simulink model "LeTronJames_Assignment2"  (R2022a)
settings: Solver=FixedStepAuto  StartTime=0.0  StopTime=60.0  FixedStep=1e-3  RelTol=1e-3  EnableMultiTasking=on
undefined symbols (not defined in the file): A0, A1, D0, D1, D10, D11, D12, D13, D2, D3, D4, D5, D6, D7, D8, D9, magnitude, PTA0, PTA1, PTA2, PTB2, PTB23, PTB3, PTB9, PTC16, PTC17, PTC2, PTC3, PTC4, PTD0, PTD1, PTD2, PTD3
libraries: frdmk64flib x19, etargetslib x2
settings Model: ExtModeTrigDuration=5  Creator=vinee  LastModifiedBy=yajatsharma
settings SolverCC: AlgebraicLoopSolver=TrustRegion
settings OptimizationCC: EnhancedBackFolding=on  PassReuseOutputArgsAs=Individual arguments  ZeroExternalMemoryAtStartup=off  ZeroInternalMemoryAtStartup=off  MaxStackSize=64  OptimizeBlockOrder=speed  DifferentSizesBufferReuse=on  OptimizationCustomize=off  EfficientTunableParamExpr=on
settings DebuggingCC: ParameterTunabilityLossMsg=error  UnconnectedInputMsg=warning  UnconnectedOutputMsg=warning  UnconnectedLineMsg=warning  SFMachineParentedDataDiag=warning
settings HardwareCC: ProdBitPerPointer=32  ProdBitPerSizeT=32  ProdBitPerPtrDiffT=32  ProdLargestAtomicInteger=Long  ProdLargestAtomicFloat=Double  ProdWordSize=32  ProdHWDeviceType=ARM Compatible->ARM Cortex
settings SFSimCC: MATLABDynamicMemAlloc=off
settings RTWCC: SystemTargetFile=ert.tlc  HardwareBoard=NXP FRDM-K64F  TLCOptions="-aInlineSetEventsForThisBaseRateFcn=TLC_FALSE -aSuppressMultiTaskScheduler=TLC_FALSE  -aRateBasedStepFcn=0"  TemplateMakefile=ert_default_tmf  Toolchain=GNU Tools for ARM Embedded Processors
settings CodeAppCC: ForceParamTrailComments=on  IgnoreCustomStorageClasses=off  OperatorAnnotations=on  SimulinkDataObjDesc=on  SFDataObjDesc=on  InsertBlockDesc=on

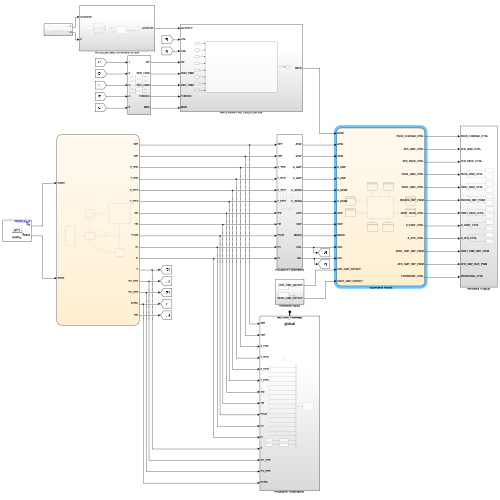
[thumbnail: Simulink's stored preview of the top-level diagram]
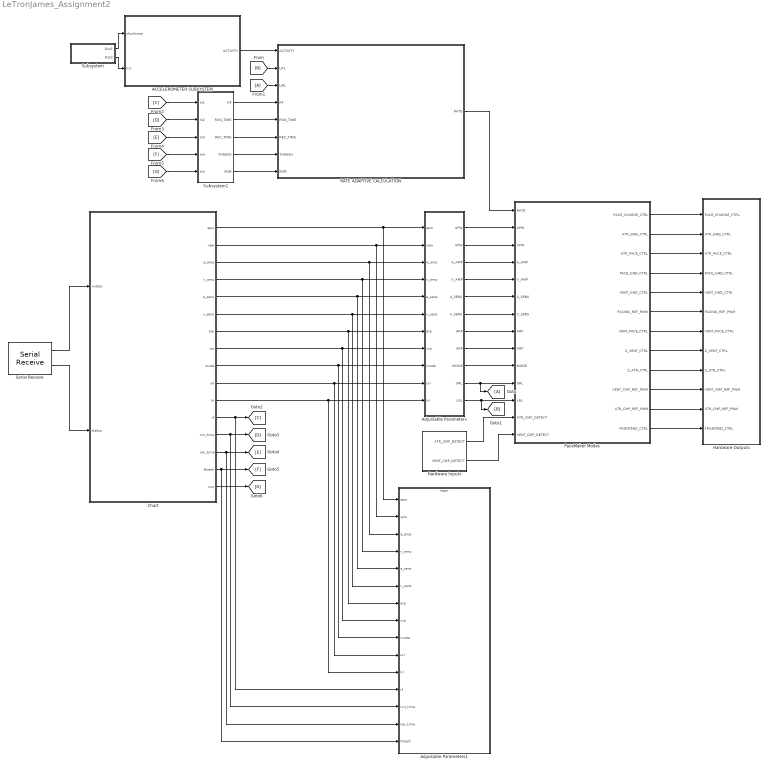
== system LeTronJames_Assignment2 ==
  ACCELEROMETER SUBSYSTEM : Subsystem
  Adjustable Parameters : Subsystem
  Adjustable Parameters1 : Subsystem
  Chart : Stateflow chart  TreatAsAtomicUnit=on
  From1 : From
  Goto : Goto
  Hardware Inputs : Subsystem
  Hardware Outputs : Subsystem
  PaceMaker Modes : Stateflow chart  TreatAsAtomicUnit=on
      settings: PortSchema="{\"entries\":[{\"content\":{\"sides\":[{\"content\":{\"connectorIds\":[\"In14\",\"In1\",\"In4\",\"In2\",\"In3\",\"In5\",\"In6\",\"In7\",\"In8\",\"In9\",\"In13\",\"In11\",\"In12\",\"In10\"]},\"type\":\"ConnectorPlacement.EquallySpacedRectSide\",\"uuid\":\"77d3ccf4-73ab-4fa0-a75b-8c1b7a05e3d5\"},{\"content\":{\"connectorIds\":[\"Out1\",\"Out2\",\"Out3\",\"Out4\",\"Out5\",\"Out6\",\"Out7\",\"Out8\",\"Out9\",\"Out10\",\"Out11\",\"Out12\"],\"side\":\"RIGHT\"},\"type\":\"ConnectorPlacement.EquallySpacedRectSide\",\"uuid\":\"3fd88102-4650-4f47-a7ab-d0892a3e0c85\"},{\"content\":{\"connectorIds\":[],\"side\":\"TOP\"},\"type\":\"ConnectorPlacement.EquallySpacedRectSide\",\"uuid\":\"24053871-acf1-4df3-bb57-3135065b83a4\"}]},\"type\":\"ConnectorPlacement.EquallySpacedConnector\",\"uuid\":\"a590c136-0049-4ce2-946f-1a46cb69b8d2\"}],\"packageUris\":[\"http://schema.mathworks.com/mf0/Connector/R2020b\"],\"version\":\"1.0\"}"
  RATE ADAPTIVE CALCULATION : Subsystem
  Serial Receive : frdmk64flib/Serial Receive  SCIModule=0  Baudrate=uint32(9600)  Parity=None  StopBits=1  HardwareFlowControl=None  ByteOrder=LittleEndian  DataType=uint8  DataLength=17  BlockingMode=off  OutputStatus=on  SampleTime=-1
  Subsystem : Subsystem
  Subsystem1 : Subsystem
  wires:
  Adjustable Parameters/1(APW) -> PaceMaker Modes/1(APW)
  PaceMaker Modes/1(PACE_CHARGE_CTRL) -> Hardware Outputs/1(PACE_CHARGE_CTRL)
  PaceMaker Modes/2(ATR_GND_CTRL) -> Hardware Outputs/2(ATR_GND_CTRL)
  PaceMaker Modes/3(ATR_PACE_CTRL) -> Hardware Outputs/3(ATR_PACE_CTRL)
  PaceMaker Modes/4(PACE_GND_CTRL) -> Hardware Outputs/4(PACE_GND_CTRL)
  PaceMaker Modes/5(VENT_GND_CTRL) -> Hardware Outputs/5(VENT_GND_CTRL)
  PaceMaker Modes/6(PACING_REF_PWM) -> Hardware Outputs/6(PACING_REF_PWM)
  PaceMaker Modes/7(VENT_PACE_CTRL) -> Hardware Outputs/7(VENT_PACE_CTRL)
  PaceMaker Modes/8(Z_VENT_CTRL) -> Hardware Outputs/8(Z_VENT_CTRL)
  PaceMaker Modes/9(Z_ATR_CTRL) -> Hardware Outputs/9(Z_ATR_CTRL)
  Hardware Inputs/2(VENT_CMP_DETECT) -> PaceMaker Modes/10(VENT_CMP_DETECT)
  Hardware Inputs/1(ATR_CMP_DETECT) -> PaceMaker Modes/12(ATR_CMP_DETECT)
  PaceMaker Modes/10(VENT_CMP_REF_PWM) -> Hardware Outputs/10(VENT_CMP_REF_PWM)
  PaceMaker Modes/11(ATR_CMP_REF_PWM) -> Hardware Outputs/11(ATR_CMP_REF_PWM)
  Adjustable Parameters/2(VPW) -> PaceMaker Modes/4(VPW)
  Adjustable Parameters/3(A_AMP) -> PaceMaker Modes/2(A_AMP)
  Adjustable Parameters/4(V_AMP) -> PaceMaker Modes/3(V_AMP)
  Adjustable Parameters/5(A_SENS) -> PaceMaker Modes/5(A_SENS)
  Adjustable Parameters/6(V_SENS) -> PaceMaker Modes/6(V_SENS)
  Adjustable Parameters/7(ARP) -> PaceMaker Modes/7(ARP)
  Adjustable Parameters/8(VRP) -> PaceMaker Modes/8(VRP)
  Adjustable Parameters/9(MODE) -> PaceMaker Modes/9(MODE)
  Adjustable Parameters/10(URL) -> Goto/1, PaceMaker Modes/13(URL)
  Adjustable Parameters/11(LRL) -> [B], PaceMaker Modes/11(LRL)
  Subsystem/1(Out1) -> ACCELEROMETER SUBSYSTEM/1(chunksize)
  Subsystem/2(Out2) -> ACCELEROMETER SUBSYSTEM/2(In1)
  [B] -> RATE ADAPTIVE CALCULATION/2(LRL)
  From1/1 -> RATE ADAPTIVE CALCULATION/3(URL)
  ACCELEROMETER SUBSYSTEM/1(ACTIVITY) -> RATE ADAPTIVE CALCULATION/1(ACTIVITY)
  RATE ADAPTIVE CALCULATION/1(RATE) -> PaceMaker Modes/14(RATE)
  Subsystem1/3(REC_TIME) -> RATE ADAPTIVE CALCULATION/6(REC_TIME)
  Subsystem1/2(RXN_TIME) -> RATE ADAPTIVE CALCULATION/5(RXN_TIME)
  Subsystem1/1(RF) -> RATE ADAPTIVE CALCULATION/4(RF)
  Subsystem1/4(THRESH) -> RATE ADAPTIVE CALCULATION/7(THRESH)
  Subsystem1/5(MSR) -> RATE ADAPTIVE CALCULATION/8(MSR)
  Chart/12(rf) -> Adjustable Parameters1/12(rf), [C]
  Chart/13(rxn_time) -> Adjustable Parameters1/13(rxn_time), [D]
  Serial Receive/1 -> Chart/1(rxdata)
  Chart/14(rec_time) -> Adjustable Parameters1/14(rec_time), [E]
  Serial Receive/2 -> Chart/2(status)
  Chart/15(thresh) -> Adjustable Parameters1/15(thresh), [F]
  [C] -> Subsystem1/1(In1)
  [E] -> Subsystem1/3(In3)
  [F] -> Subsystem1/4(In4)
  [D] -> Subsystem1/2(In2)
  [G] -> Subsystem1/5(In5)
  Chart/11(lrl) -> Adjustable Parameters1/11(lrl), Adjustable Parameters/11(lrl)
  Chart/10(url) -> Adjustable Parameters1/10(url), Adjustable Parameters/10(url)
  Chart/9(mode) -> Adjustable Parameters1/9(mode), Adjustable Parameters/9(mode)
  Chart/8(vrp) -> Adjustable Parameters1/8(vrp), Adjustable Parameters/8(vrp)
  Chart/7(arp) -> Adjustable Parameters1/7(arp), Adjustable Parameters/7(arp)
  Chart/6(v_sens) -> Adjustable Parameters1/6(v_sens), Adjustable Parameters/6(v_sens)
  Chart/5(a_sens) -> Adjustable Parameters1/5(a_sens), Adjustable Parameters/5(a_sens)
  Chart/4(v_amp) -> Adjustable Parameters1/4(v_amp), Adjustable Parameters/4(v_amp)
  Chart/3(a_amp) -> Adjustable Parameters1/3(a_amp), Adjustable Parameters/3(a_amp)
  Chart/2(vpw) -> Adjustable Parameters1/2(vpw), Adjustable Parameters/2(vpw)
  Chart/1(apw) -> Adjustable Parameters1/1(apw), Adjustable Parameters/1(apw)
  Chart/16(msr) -> [G]
  PaceMaker Modes/12(FRONTEND_CTRL) -> Hardware Outputs/12(FRONTEND_CTRL)

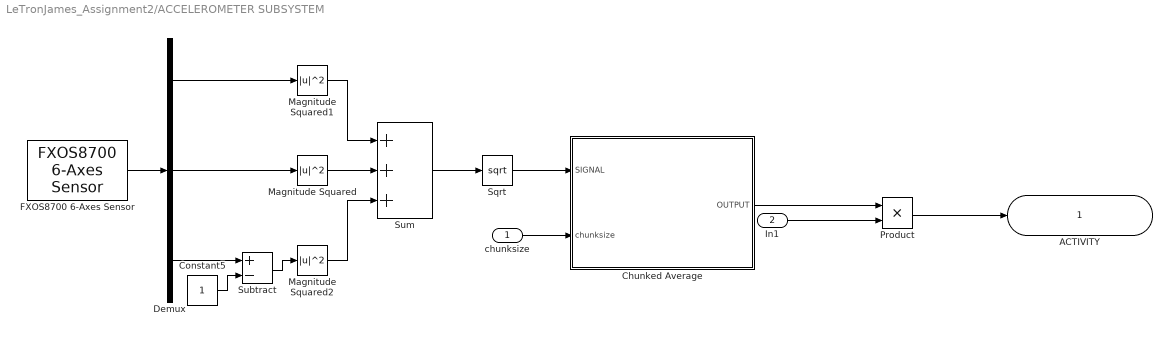
== system LeTronJames_Assignment2/ACCELEROMETER SUBSYSTEM ==
  chunksize : Inport
  In1 : Inport  Port=2
  Chunked Average : Stateflow chart  TreatAsAtomicUnit=on
  Constant5 : Constant
  Demux : Demux  Outputs=3
  FXOS8700 6-Axes Sensor : frdmk64flib/FXOS8700 6-Axes Sensor  Activesensor=Accelerometer only  ODR=800Hz  HybridODR=400Hz  Accelfullrange=-4g to +4g  SampleTime=0.01
  Magnitude Squared : Math  Operator=magnitude^2
  Magnitude Squared1 : Math  Operator=magnitude^2
  Magnitude Squared2 : Math  Operator=magnitude^2
  Product : Product  OutDataTypeStr=uint16
  Sqrt : Sqrt  IntermediateResultsDataTypeStr=double
  Subtract : Sum  Inputs=+-
  Sum : Sum  Inputs=+++
  ACTIVITY : Outport
  wires:
  Chunked Average/1(OUTPUT) -> Product/1
  Sum/1 -> Sqrt/1
  Demux/1 -> Magnitude Squared1/1
  FXOS8700 6-Axes Sensor/1 -> Demux/1
  Demux/2 -> Magnitude Squared/1
  Subtract/1 -> Magnitude Squared2/1
  Constant5/1 -> Subtract/2
  Magnitude Squared/1 -> Sum/2
  Magnitude Squared2/1 -> Sum/3
  Magnitude Squared1/1 -> Sum/1
  Demux/3 -> Subtract/1
  In1/1 -> Product/2
  Product/1 -> ACTIVITY/1
  chunksize/1 -> Chunked Average/2(chunksize)
  Sqrt/1 -> Chunked Average/1(SIGNAL)

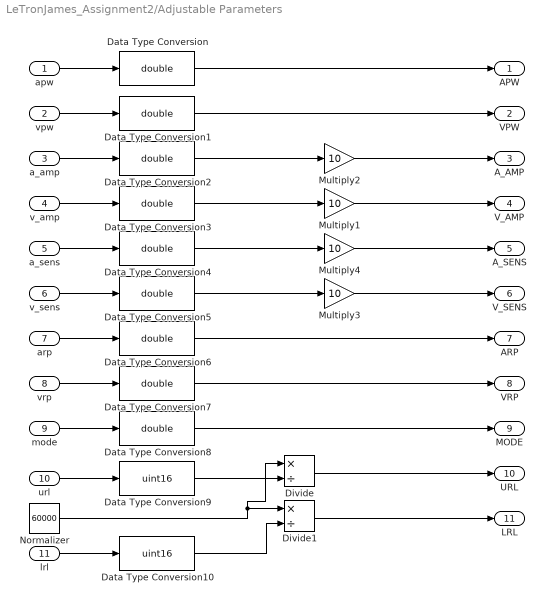
== system LeTronJames_Assignment2/Adjustable Parameters ==
  apw : Inport
  vpw : Inport  Port=2
  a_amp : Inport  Port=3
  v_amp : Inport  Port=4
  a_sens : Inport  Port=5
  v_sens : Inport  Port=6
  arp : Inport  Port=7
  vrp : Inport  Port=8
  mode : Inport  Port=9
  url : Inport  Port=10
  lrl : Inport  Port=11
  Data Type Conversion{,1..8} (9 alike) : DataTypeConversion  OutDataTypeStr=double  SaturateOnIntegerOverflow=off  RndMeth=Floor
  Data Type Conversion10 : DataTypeConversion  OutDataTypeStr=uint16  SaturateOnIntegerOverflow=off  RndMeth=Floor
  Data Type Conversion9 : DataTypeConversion  OutDataTypeStr=uint16  SaturateOnIntegerOverflow=off  RndMeth=Floor
  Divide : Product  Inputs=*/
  Divide1 : Product  Inputs=*/
  Multiply{1..4} (4 alike) : Gain  Gain=10
  Normalizer : Constant  Value=60000  OutDataTypeStr=uint16
  APW : Outport
  VPW : Outport  Port=2
  A_AMP : Outport  Port=3
  V_AMP : Outport  Port=4
  A_SENS : Outport  Port=5
  V_SENS : Outport  Port=6
  ARP : Outport  Port=7
  VRP : Outport  Port=8
  MODE : Outport  Port=9
  URL : Outport  Port=10
  LRL : Outport  Port=11
  wires:
  Multiply1/1 -> V_AMP/1
  Normalizer/1 -> Divide/1, Divide1/1
  Divide/1 -> URL/1
  Multiply2/1 -> A_AMP/1
  Divide1/1 -> LRL/1
  vpw/1 -> Data Type Conversion1/1
  apw/1 -> Data Type Conversion/1
  a_amp/1 -> Data Type Conversion2/1
  v_amp/1 -> Data Type Conversion3/1
  a_sens/1 -> Data Type Conversion4/1
  v_sens/1 -> Data Type Conversion5/1
  arp/1 -> Data Type Conversion6/1
  vrp/1 -> Data Type Conversion7/1
  mode/1 -> Data Type Conversion8/1
  lrl/1 -> Data Type Conversion10/1
  url/1 -> Data Type Conversion9/1
  Data Type Conversion/1 -> APW/1
  Data Type Conversion1/1 -> VPW/1
  Data Type Conversion2/1 -> Multiply2/1
  Data Type Conversion3/1 -> Multiply1/1
  Data Type Conversion6/1 -> ARP/1
  Data Type Conversion7/1 -> VRP/1
  Data Type Conversion8/1 -> MODE/1
  Data Type Conversion9/1 -> Divide/2
  Data Type Conversion10/1 -> Divide1/2
  Data Type Conversion5/1 -> Multiply3/1
  Data Type Conversion4/1 -> Multiply4/1
  Multiply3/1 -> V_SENS/1
  Multiply4/1 -> A_SENS/1

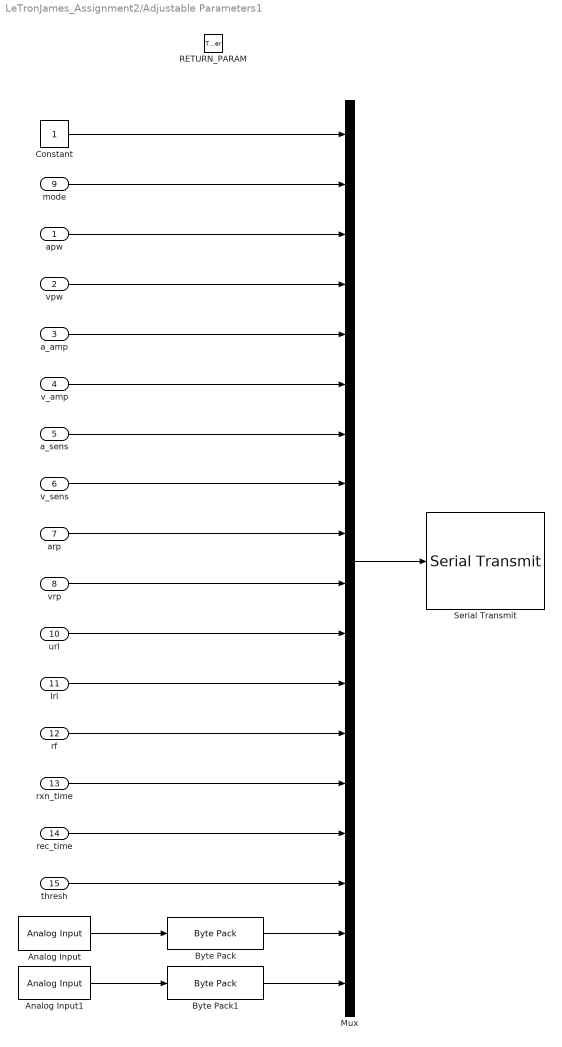
== system LeTronJames_Assignment2/Adjustable Parameters1 ==
  apw : Inport
  vpw : Inport  Port=2
  a_amp : Inport  Port=3
  v_amp : Inport  Port=4
  a_sens : Inport  Port=5
  v_sens : Inport  Port=6
  arp : Inport  Port=7
  vrp : Inport  Port=8
  mode : Inport  Port=9
  url : Inport  Port=10
  lrl : Inport  Port=11
  rf : Inport  Port=12
  rxn_time : Inport  Port=13
  rec_time : Inport  Port=14
  thresh : Inport  Port=15
  RETURN_PARAM : TriggerPort  TriggerType=function-call  IsSimulinkFunction=on  FunctionName=RETURN_PARAM  VariantControl=Variant
  Analog Input : frdmk64flib/Analog Input  Whichpin=PTB2 (A0)  SampleTime=-1
  Analog Input1 : frdmk64flib/Analog Input  Whichpin=PTB3 (A1)  SampleTime=-1
  Byte Pack : etargetslib/Byte Pack  datatypes={'double'}  byteAlign=1
  Byte Pack1 : etargetslib/Byte Pack  datatypes={'double'}  byteAlign=1
  Constant : Constant  OutDataTypeStr=uint8
  Mux : Mux  Inputs=18
  Serial Transmit : frdmk64flib/Serial Transmit  SCIModule=0  Baudrate=uint32(9600)  Parity=None  StopBits=1  HardwareFlowControl=None  ByteOrder=LittleEndian  BlockingMode=on  OutputStatus=off
  wires:
  Mux/1 -> Serial Transmit/1
  Analog Input/1 -> Byte Pack/1
  Analog Input1/1 -> Byte Pack1/1
  Byte Pack/1 -> Mux/17
  Constant/1 -> Mux/1
  mode/1 -> Mux/2
  thresh/1 -> Mux/16
  rec_time/1 -> Mux/15
  rxn_time/1 -> Mux/14
  rf/1 -> Mux/13
  lrl/1 -> Mux/12
  url/1 -> Mux/11
  vrp/1 -> Mux/10
  arp/1 -> Mux/9
  v_sens/1 -> Mux/8
  a_sens/1 -> Mux/7
  v_amp/1 -> Mux/6
  a_amp/1 -> Mux/5
  vpw/1 -> Mux/4
  apw/1 -> Mux/3
  Byte Pack1/1 -> Mux/18

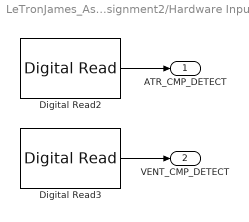
== system LeTronJames_Assignment2/Hardware Inputs ==
  Digital Read2 : frdmk64flib/Digital Read  Whichpin=PTC16 (D0)  SampleTime=-1
  Digital Read3 : frdmk64flib/Digital Read  Whichpin=PTC17 (D1)  SampleTime=-1
  ATR_CMP_DETECT : Outport
  VENT_CMP_DETECT : Outport  Port=2
  wires:
  Digital Read3/1 -> VENT_CMP_DETECT/1
  Digital Read2/1 -> ATR_CMP_DETECT/1

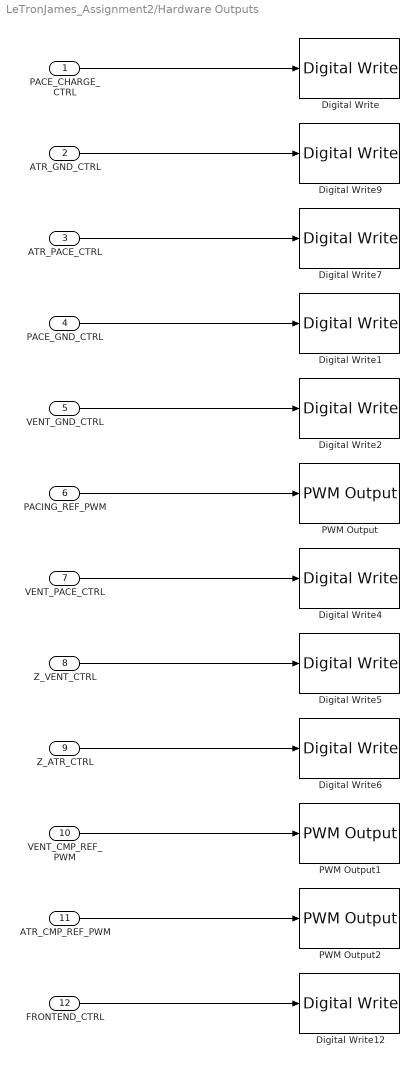
== system LeTronJames_Assignment2/Hardware Outputs ==
  PACE_CHARGE_CTRL : Inport
  ATR_GND_CTRL : Inport  Port=2
  ATR_PACE_CTRL : Inport  Port=3
  PACE_GND_CTRL : Inport  Port=4
  VENT_GND_CTRL : Inport  Port=5
  PACING_REF_PWM : Inport  Port=6
  VENT_PACE_CTRL : Inport  Port=7
  Z_VENT_CTRL : Inport  Port=8
  Z_ATR_CTRL : Inport  Port=9
  VENT_CMP_REF_PWM : Inport  Port=10
  ATR_CMP_REF_PWM : Inport  Port=11
  FRONTEND_CTRL : Inport  Port=12
  Digital Write : frdmk64flib/Digital Write  Whichpin=PTB9 (D2)
  Digital Write1 : frdmk64flib/Digital Write  Whichpin=PTD0 (D10)
  Digital Write12 : frdmk64flib/Digital Write  Whichpin=PTD1 (D13)
  Digital Write2 : frdmk64flib/Digital Write  Whichpin=PTD3 (D12)
  Digital Write4 : frdmk64flib/Digital Write  Whichpin=PTC4 (D9)
  Digital Write5 : frdmk64flib/Digital Write  Whichpin=PTC3 (D7)
  Digital Write6 : frdmk64flib/Digital Write  Whichpin=PTB23 (D4)
  Digital Write7 : frdmk64flib/Digital Write  Whichpin=PTA0 (D8)
  Digital Write9 : frdmk64flib/Digital Write  Whichpin=PTD2 (D11)
  PWM Output : frdmk64flib/PWM Output  Whichpin=PTA2 (D5)  InitialFrequency=2000  InitialDutyCycle=0
  PWM Output1 : frdmk64flib/PWM Output  Whichpin=PTA1 (D3)  InitialFrequency=2000  InitialDutyCycle=0
  PWM Output2 : frdmk64flib/PWM Output  Whichpin=PTC2 (D6)  InitialFrequency=2000  InitialDutyCycle=0
  wires:
  PACE_CHARGE_CTRL/1 -> Digital Write/1
  ATR_GND_CTRL/1 -> Digital Write9/1
  ATR_PACE_CTRL/1 -> Digital Write7/1
  PACE_GND_CTRL/1 -> Digital Write1/1
  VENT_GND_CTRL/1 -> Digital Write2/1
  PACING_REF_PWM/1 -> PWM Output/1
  VENT_PACE_CTRL/1 -> Digital Write4/1
  Z_VENT_CTRL/1 -> Digital Write5/1
  Z_ATR_CTRL/1 -> Digital Write6/1
  VENT_CMP_REF_PWM/1 -> PWM Output1/1
  ATR_CMP_REF_PWM/1 -> PWM Output2/1
  FRONTEND_CTRL/1 -> Digital Write12/1

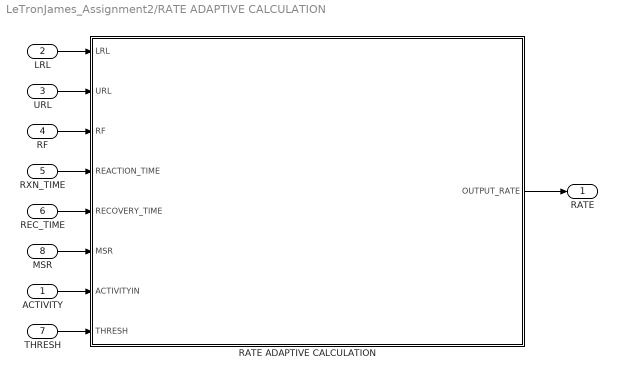
== system LeTronJames_Assignment2/RATE ADAPTIVE CALCULATION ==
  ACTIVITY : Inport
  LRL : Inport  Port=2
  URL : Inport  Port=3
  RF : Inport  Port=4
  RXN_TIME : Inport  Port=5
  REC_TIME : Inport  Port=6
  THRESH : Inport  Port=7
  MSR : Inport  Port=8
  RATE ADAPTIVE CALCULATION : Stateflow chart  TreatAsAtomicUnit=on
      settings: PortSchema="{\"entries\":[{\"content\":{\"sides\":[{\"content\":{\"connectorIds\":[\"In1\",\"In2\",\"In4\",\"In5\",\"In6\",\"In7\",\"In8\",\"In3\"]},\"type\":\"ConnectorPlacement.EquallySpacedRectSide\",\"uuid\":\"0d1f97db-42d8-44a9-a405-14d2ab31c0c4\"},{\"content\":{\"connectorIds\":[\"Out1\"],\"side\":\"RIGHT\"},\"type\":\"ConnectorPlacement.EquallySpacedRectSide\",\"uuid\":\"c963fb94-52d4-44e1-a6a0-ca4b2ff51e25\"},{\"content\":{\"connectorIds\":[],\"side\":\"TOP\"},\"type\":\"ConnectorPlacement.EquallySpacedRectSide\",\"uuid\":\"fb7430b2-7c41-4258-9d6d-2418378c9820\"}]},\"type\":\"ConnectorPlacement.EquallySpacedConnector\",\"uuid\":\"11cb7a60-c1bd-4ee9-9a44-3319425add7f\"}],\"packageUris\":[\"http://schema.mathworks.com/mf0/Connector/R2020b\"],\"version\":\"1.0\"}"
  RATE : Outport  OutDataTypeStr=uint16
  wires:
  LRL/1 -> RATE ADAPTIVE CALCULATION/1(LRL)
  RXN_TIME/1 -> RATE ADAPTIVE CALCULATION/5(REACTION_TIME)
  REC_TIME/1 -> RATE ADAPTIVE CALCULATION/6(RECOVERY_TIME)
  THRESH/1 -> RATE ADAPTIVE CALCULATION/3(THRESH)
  RF/1 -> RATE ADAPTIVE CALCULATION/4(RF)
  RATE ADAPTIVE CALCULATION/1(OUTPUT_RATE) -> RATE/1
  ACTIVITY/1 -> RATE ADAPTIVE CALCULATION/8(ACTIVITYIN)
  URL/1 -> RATE ADAPTIVE CALCULATION/2(URL)
  MSR/1 -> RATE ADAPTIVE CALCULATION/7(MSR)

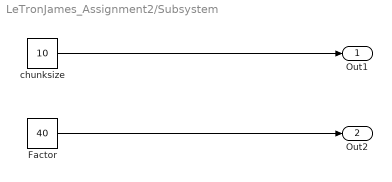
== system LeTronJames_Assignment2/Subsystem ==
  Factor : Constant  Value=40
  chunksize : Constant  Value=10
  Out1 : Outport
  Out2 : Outport  Port=2
  wires:
  chunksize/1 -> Out1/1
  Factor/1 -> Out2/1

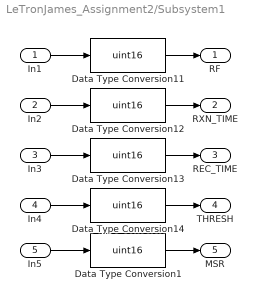
== system LeTronJames_Assignment2/Subsystem1 ==
  In1 : Inport
  In2 : Inport  Port=2
  In3 : Inport  Port=3
  In4 : Inport  Port=4
  In5 : Inport  Port=5
  Data Type Conversion{1,11..14} (5 alike) : DataTypeConversion  OutDataTypeStr=uint16  SaturateOnIntegerOverflow=off  RndMeth=Floor
  RF : Outport
  RXN_TIME : Outport  Port=2
  REC_TIME : Outport  Port=3
  THRESH : Outport  Port=4
  MSR : Outport  Port=5
  wires:
  In4/1 -> Data Type Conversion14/1
  In1/1 -> Data Type Conversion11/1
  In2/1 -> Data Type Conversion12/1
  In3/1 -> Data Type Conversion13/1
  Data Type Conversion11/1 -> RF/1
  Data Type Conversion12/1 -> RXN_TIME/1
  Data Type Conversion13/1 -> REC_TIME/1
  Data Type Conversion14/1 -> THRESH/1
  Data Type Conversion1/1 -> MSR/1
  In5/1 -> Data Type Conversion1/1

== stateflow chart LeTronJames_Assignment2/Chart ==
  state SET_PARAM
    entry:
    mode = rxdata(3);
    apw = rxdata(4);
    vpw = rxdata(5);
    a_amp = rxdata(6);
    v_amp = rxdata(7);
    a_sens = rxdata(8);
    v_sens = rxdata(9);
    arp = rxdata(10);
    vrp = rxdata(11);
    url = rxdata(12);
    lrl = rxdata(13);
    rf = rxdata(14);
    rxn_time = rxdata(15);
    rec_time = rxdata(16);
    thresh = rxdata(17);
  state SEND_EGRAM
    entry:
    RETURN_PARAM()
  state INITIAL
    entry:
    mode = 1;
    apw = 5;
    vpw = 5;
    a_amp = 10;
    v_amp = 5;
    a_sens = 6;
    v_sens = 6;
    arp = 100;
    vrp = 150;
    url = 120;
    lrl = 60;
    rf = 8;
    rxn_time = 30;
    rec_time = 5;
    thresh = 120;
    msr = 120;
  state STANDBY
  state SEND_PARAMS
    entry:
    RETURN_PARAM()
  SET_PARAM -> SEND_EGRAM
  SEND_EGRAM -> STANDBY
  (junction 22) -> SET_PARAM [order 1] : [rxdata(2) == 0]
  (default) -> INITIAL
  (junction 20) -> STANDBY [order 2]
  INITIAL -> STANDBY
  STANDBY -> (junction 20) : [status == 0]
  (junction 20) -> (junction 22) [order 1] : [rxdata(1) ==  1]
  (junction 22) -> SEND_PARAMS [order 2] : [rxdata(2) == 1]
  SEND_PARAMS -> STANDBY
  data: apw output uint8; vpw output uint8; a_amp output uint8; v_amp output uint8; a_sens output uint8; v_sens output uint8; arp output uint8; vrp output uint8; mode output uint8; url output uint8; lrl output uint8; rf output uint8; rxn_time output uint8; rec_time output uint8; thresh output uint8; rxdata input; status input; msr output uint8

== stateflow chart LeTronJames_Assignment2/ACCELEROMETER SUBSYSTEM/Chunked Average ==
  state OUTPUT_STATE
    entry:
    total = total/COUNTER;
    OUTPUT = total;
    %computes the average to smooth out signal
  state COUNTER_STATE
    entry:
    total = total + SIGNAL;
    COUNTER = COUNTER + 1;
    %Finds the running total of the signals
  (default) -> COUNTER_STATE : {COUNTER=0, total=0}
  OUTPUT_STATE -> COUNTER_STATE : {COUNTER = 0, total = 0}
  COUNTER_STATE -> OUTPUT_STATE [order 1] : [COUNTER >= chunksize]
  COUNTER_STATE -> COUNTER_STATE [order 2] : [COUNTER < chunksize]
  data: COUNTER local; total local; SIGNAL input; OUTPUT output; chunksize input

== stateflow chart LeTronJames_Assignment2/PaceMaker Modes ==
  state AOOR %This is the chart for the AOOR mode
    % All of the values outside here are unchanging for charging and discharging
    entry:
    Z_ATR_CTRL = false;
    Z_VENT_CTRL =false;
    VENT_GND_CTRL = false;
    VENT_PACE_CTRL =false;
    PACING_REF_PWM = A_AMP;
    ADAPTIVERATE = 60000/RATE;
    FRONTEND_CTRL = true;
    %steps are in the correct order for safety
    %discharged for duration of pulse width
    %ADAPTIVERATE is used to account for changes in pulsing rate due to the acceleration of the pacemaker
    state DISCHARGE_STATE
      entry:
      PACE_CHARGE_CTRL = false;
      ATR_PACE_CTRL = true;
      ATR_GND_CTRL = false;
      PACE_GND_CTRL = true;
      ADAPTIVERATE = 60000/RATE;
    state CHARGE_STATE
      entry:
      ATR_PACE_CTRL = false;
      ATR_GND_CTRL = true;
      PACE_CHARGE_CTRL =false;
      PACE_GND_CTRL = false;
    (default) -> AOOR.CHARGE_STATE
    AOOR.DISCHARGE_STATE -> AOOR.CHARGE_STATE : after(APW, msec)
    AOOR.CHARGE_STATE -> AOOR.DISCHARGE_STATE : after(ADAPTIVERATE - APW ,msec)
  state AAIR%This is the chart for the AAIR mode
    % All of the values outside here are unchanging for charging, discharging, and sensing
    entry:
    Z_ATR_CTRL = false;
    Z_VENT_CTRL =false;
    VENT_GND_CTRL = false;
    VENT_PACE_CTRL =false;
    PACE_GND_CTRL = true;
    PACING_REF_PWM = A_AMP;
    ATR_CMP_REF_PWM = A_SENS;
    FRONTEND_CTRL = true;
    ADAPTIVERATE = 60000/RATE;
    %steps are in the correct order for safety
    %discharged depending on wether natural pulse is sensed or not
    %requires the sensing state to wait and detect
    %ADAPTIVERATE is meant to change the pacing rate based on the rate
    %calculation that is inputted as RATE
    state DISCHARGE_STATE
      entry:
      ATR_PACE_CTRL = true;
      ATR_GND_CTRL = false;
      PACE_CHARGE_CTRL = false;
      ADAPTIVERATE = 60000/RATE;
    state CHARGE_STATE
      entry:
      ATR_PACE_CTRL = false;
      ATR_GND_CTRL = true;
      PACE_CHARGE_CTRL =true;
      ADAPTIVERATE = 60000/RATE;
    state ATR_SENSING
      entry:
      ATR_PACE_CTRL = false;
      ATR_GND_CTRL = true;
      PACE_CHARGE_CTRL =true;
      ADAPTIVERATE = 60000/RATE;
    (default) -> AAIR%This.CHARGE_STATE
    AAIR%This.CHARGE_STATE -> AAIR%This.DISCHARGE_STATE [order 2] : after(ADAPTIVERATE-ARP-APW, msec)
    AAIR%This.ATR_SENSING -> AAIR%This.CHARGE_STATE : after(ARP,msec)
    AAIR%This.CHARGE_STATE -> AAIR%This.ATR_SENSING [order 1] : [ATR_CMP_DETECT == true]
    AAIR%This.DISCHARGE_STATE -> AAIR%This.ATR_SENSING : after(APW ,msec)
  state AOO %This is the chart for the AOO mode
    % All of the values outside here are unchanging for charging and discharging
    entry:
    Z_ATR_CTRL = false;
    Z_VENT_CTRL =false;
    VENT_GND_CTRL = false;
    VENT_PACE_CTRL =false;
    PACING_REF_PWM = A_AMP;
    FRONTEND_CTRL = true;
    %steps are in the correct order for safety
    %discharged for duration of pulse width
    state DISCHARGE_STATE
      entry:
      PACE_CHARGE_CTRL = false;
      ATR_PACE_CTRL = true;
      ATR_GND_CTRL = false;
      PACE_GND_CTRL = true;
    state CHARGE_STATE
      entry:
      ATR_PACE_CTRL = false;
      ATR_GND_CTRL = true;
      PACE_CHARGE_CTRL =false;
      PACE_GND_CTRL = false;
    (default) -> AOO.CHARGE_STATE
    AOO.DISCHARGE_STATE -> AOO.CHARGE_STATE : after(APW, msec)
    AOO.CHARGE_STATE -> AOO.DISCHARGE_STATE : after(LRL - APW ,msec)
  state MODE_SELECTOR
    entry:
    %This state is to switch between modes
    %resets all the variables for safety
    ATR_PACE_CTRL = false;
    ATR_GND_CTRL = false;
    VENT_GND_CTRL = false;
    VENT_PACE_CTRL = false;
    Z_ATR_CTRL = false;
    Z_VENT_CTRL = false;
    ATR_CMP_REF_PWM = 0;
    VENT_CMP_REF_PWM= 0;
    PACE_GND_CTRL = false;
    PACE_CHARGE_CTRL = false;
    FRONTEND_CTRL = false;
    ADAPTIVERATE = 60000/RATE;
  state VOO%This is the chart for the VOO mode
    % All of the values outside here are unchanging for charging and discharging
    entry:
    Z_ATR_CTRL = false;
    Z_VENT_CTRL =false;
    ATR_GND_CTRL = false;
    ATR_PACE_CTRL = false;
    PACING_REF_PWM = V_AMP;
    FRONTEND_CTRL = true;
    %steps are in the correct order for safety
    %discharged for duration of the pulse width
    state DISCHARGE_STATE
      entry:
      PACE_CHARGE_CTRL = false;
      VENT_PACE_CTRL = true;
      VENT_GND_CTRL = false;
      PACE_GND_CTRL = true;
    state CHARGE_STATE
      entry:
      VENT_PACE_CTRL = false;
      VENT_GND_CTRL = true;
      PACE_CHARGE_CTRL = true;
      PACE_GND_CTRL = false;
    (default) -> VOO%This.CHARGE_STATE
    VOO%This.DISCHARGE_STATE -> VOO%This.CHARGE_STATE : after(VPW, msec)
    VOO%This.CHARGE_STATE -> VOO%This.DISCHARGE_STATE : after(LRL - VPW ,msec)
  state VVI%This is the chart for the VVI mode
    % All of the values outside here are unchanging for charging, discharging, and sensing
    entry:
    Z_ATR_CTRL = false;
    Z_VENT_CTRL = false;
    ATR_GND_CTRL = false;
    ATR_PACE_CTRL = false;
    PACE_GND_CTRL = true;
    PACING_REF_PWM = V_AMP;
    VENT_CMP_REF_PWM = V_SENS;
    FRONTEND_CTRL = true;
    %steps are in the correct order for safety
    %discharged depending on wether natural pulse is sensed or not
    %requires the sensing state to wait and detect
    state DISCHARGE_STATE
      entry:
      VENT_PACE_CTRL = true;
      VENT_GND_CTRL = false;
      PACE_CHARGE_CTRL = false;
    state CHARGE_STATE
      entry:
      VENT_PACE_CTRL = false;
      VENT_GND_CTRL = true;
      PACE_CHARGE_CTRL =true;
    state VENT_SENSING
      entry:
      VENT_PACE_CTRL = false;
      VENT_GND_CTRL = true;
      PACE_CHARGE_CTRL =true;
    (default) -> VVI%This.CHARGE_STATE
    VVI%This.CHARGE_STATE -> VVI%This.DISCHARGE_STATE [order 2] : after(LRL-VRP-VPW, msec)
    VVI%This.VENT_SENSING -> VVI%This.CHARGE_STATE : after(VRP,msec)
    VVI%This.CHARGE_STATE -> VVI%This.VENT_SENSING [order 1] : [VENT_CMP_DETECT == true]
    VVI%This.DISCHARGE_STATE -> VVI%This.VENT_SENSING : after(VPW ,msec)
  state AAI%This is the chart for the AAI mode
    % All of the values outside here are unchanging for charging, discharging, and sensing
    entry:
    Z_ATR_CTRL = false;
    Z_VENT_CTRL =false;
    VENT_GND_CTRL = false;
    VENT_PACE_CTRL =false;
    PACE_GND_CTRL = true;
    PACING_REF_PWM = A_AMP;
    ATR_CMP_REF_PWM = A_SENS;
    FRONTEND_CTRL = true;
    %steps are in the correct order for safety
    %discharged depending on wether natural pulse is sensed or not
    %requires the sensing state to wait and detect
    state DISCHARGE_STATE
      entry:
      ATR_PACE_CTRL = true;
      ATR_GND_CTRL = false;
      PACE_CHARGE_CTRL = false;
    state CHARGE_STATE
      entry:
      ATR_PACE_CTRL = false;
      ATR_GND_CTRL = true;
      PACE_CHARGE_CTRL =true;
    state ATR_SENSING
      entry:
      ATR_PACE_CTRL = false;
      ATR_GND_CTRL = true;
      PACE_CHARGE_CTRL =true;
    (default) -> AAI%This.CHARGE_STATE
    AAI%This.CHARGE_STATE -> AAI%This.DISCHARGE_STATE [order 2] : after(LRL-ARP-APW, msec)
    AAI%This.ATR_SENSING -> AAI%This.CHARGE_STATE : after(ARP,msec)
    AAI%This.CHARGE_STATE -> AAI%This.ATR_SENSING [order 1] : [ATR_CMP_DETECT == true]
    AAI%This.DISCHARGE_STATE -> AAI%This.ATR_SENSING : after(APW ,msec)
  state VOOR%This is the chart for the VOOR mode
    % All of the values outside here are unchanging for charging and discharging
    entry:
    Z_ATR_CTRL = false;
    Z_VENT_CTRL =false;
    ATR_GND_CTRL = false;
    ATR_PACE_CTRL = false;
    PACING_REF_PWM = V_AMP;
    ADAPTIVERATE = 60000/RATE;
    FRONTEND_CTRL = true;
    %steps are in the correct order for safety
    %discharged for duration of the pulse width
    %The ADAPTIVERATE is to account for the changes in pulsing rate due to the acceleration data
    state DISCHARGE_STATE
      entry:
      PACE_CHARGE_CTRL = false;
      VENT_PACE_CTRL = true;
      VENT_GND_CTRL = false;
      PACE_GND_CTRL = true;
      ADAPTIVERATE = 60000/RATE;
    state CHARGE_STATE
      entry:
      VENT_PACE_CTRL = false;
      VENT_GND_CTRL = true;
      PACE_CHARGE_CTRL = true;
      PACE_GND_CTRL = false;
    (default) -> VOOR%This.CHARGE_STATE
    VOOR%This.DISCHARGE_STATE -> VOOR%This.CHARGE_STATE : after(VPW, msec)
    VOOR%This.CHARGE_STATE -> VOOR%This.DISCHARGE_STATE : after(ADAPTIVERATE - VPW ,msec)
  state VVIR
    %This is the chart for the VVIR mode
    % All of the values outside here are unchanging for charging, discharging, and sensing
    entry:
    Z_ATR_CTRL = false;
    Z_VENT_CTRL = false;
    ATR_GND_CTRL = false;
    ATR_PACE_CTRL = false;
    PACE_GND_CTRL = true;
    PACING_REF_PWM = V_AMP;
    VENT_CMP_REF_PWM = V_SENS;
    FRONTEND_CTRL = true;
    ADAPTIVERATE = 60000/RATE;
    %steps are in the correct order for safety
    %discharged depending on wether natural pulse is sensed or not
    %requires the sensing state to wait and detect
    %ADAPTIVERATE is to account for the changes in pacing rate
    %due to the accelerometer
    state DISCHARGE_STATE
      entry:
      VENT_PACE_CTRL = true;
      VENT_GND_CTRL = false;
      PACE_CHARGE_CTRL = false;
      ADAPTIVERATE = 60000/RATE;
    state CHARGE_STATE
      entry:
      VENT_PACE_CTRL = false;
      VENT_GND_CTRL = true;
      PACE_CHARGE_CTRL =true;
      ADAPTIVERATE = 60000/RATE;
    state VENT_SENSING
      entry:
      VENT_PACE_CTRL = false;
      VENT_GND_CTRL = true;
      PACE_CHARGE_CTRL =true;
      ADAPTIVERATE = 60000/RATE;
    (default) -> VVIR.CHARGE_STATE
    VVIR.CHARGE_STATE -> VVIR.DISCHARGE_STATE [order 2] : after(ADAPTIVERATE-VRP-VPW, msec)
    VVIR.VENT_SENSING -> VVIR.CHARGE_STATE : after(VRP,msec)
    VVIR.DISCHARGE_STATE -> VVIR.VENT_SENSING : after(VPW ,msec)
    VVIR.CHARGE_STATE -> VVIR.VENT_SENSING [order 1] : [VENT_CMP_DETECT == true]
  (default) -> MODE_SELECTOR
  AAIR%This is the chart for the AAIR mode -> MODE_SELECTOR : [MODE ~=7]
  MODE_SELECTOR -> AAIR%This is the chart for the AAIR mode [order 7] : [MODE==7]
  AOOR %This is the chart for the AOOR mode -> MODE_SELECTOR : [MODE~=5 ]
  MODE_SELECTOR -> AOOR %This is the chart for the AOOR mode [order 5] : [MODE == 5]
  MODE_SELECTOR -> AOO %This is the chart for the AOO mode [order 1] : [MODE == 1]
  MODE_SELECTOR -> VOO%This is the chart for the VOO mode [order 2] : [MODE == 2]
  VOO%This is the chart for the VOO mode -> MODE_SELECTOR : [MODE ~= 2]
  AOO %This is the chart for the AOO mode -> MODE_SELECTOR : [MODE~=1 ]
  MODE_SELECTOR -> AAI%This is the chart for the AAI mode [order 3] : [MODE==3]
  MODE_SELECTOR -> VVI%This is the chart for the VVI mode [order 4] : [MODE==4]
  VVI%This is the chart for the VVI mode -> MODE_SELECTOR : [MODE~=4]
  AAI%This is the chart for the AAI mode -> MODE_SELECTOR : [MODE ~=3]
  VOOR%This is the chart for the VOOR mode -> MODE_SELECTOR : [MODE ~= 6]
  MODE_SELECTOR -> VOOR%This is the chart for the VOOR mode [order 6] : [MODE == 6]
  VVIR -> MODE_SELECTOR : [MODE~=8]
  MODE_SELECTOR -> VVIR [order 8] : [MODE==8]
  data: PACE_CHARGE_CTRL output boolean; ATR_GND_CTRL output boolean; ATR_PACE_CTRL output boolean; PACE_GND_CTRL output boolean; VENT_GND_CTRL output boolean; PACING_REF_PWM output; VENT_PACE_CTRL output boolean; Z_VENT_CTRL output; Z_ATR_CTRL output; APW input; A_AMP input; V_AMP input; VPW input double; A_SENS input; V_SENS input; ARP input; VRP input; MODE input; VENT_CMP_DETECT input boolean; LRL input; ATR_CMP_DETECT input boolean; VENT_CMP_REF_PWM output double; ATR_CMP_REF_PWM output; FRONTEND_CTRL output boolean; URL input; RATE input uint16; ADAPTIVERATE local uint16; RATEin local

== stateflow chart LeTronJames_Assignment2/RATE ADAPTIVE CALCULATION/RATE ADAPTIVE CALCULATION ==
  state START
    entry:
    LRLnorm = (60000/LRL);
    URLnorm =(60000/URL);
    RATE = LRLnorm;
  state RATE_CALCULATION
    entry:
    step_reaction = (URLnorm - LRLnorm)/(REACTION_TIME*5);
    step_recovery = (URLnorm- LRLnorm)/(RECOVERY_TIME*5);
    if (RATE < TARGET)
    RATE = RATE + step_reaction;
    end
    if (RATE > TARGET)
    RATE = RATE - step_recovery;
    end
    if (RATE > URLnorm)
    RATE = URLnorm;
    end
    if (RATE < LRLnorm)
    RATE = LRLnorm;
    end
    OUTPUT_RATE = RATE;
    %OUTPUT_RATE = 500;
  state SLOPE_CALCULATION
    entry:
    %slope = ((RF)/(10*URL) * (URL - (THRESH)));
    ACTIVITY = ACTIVITYIN;
    slope = 0.75*RF;
    TARGET = slope*(ACTIVITY - THRESH) + LRLnorm;
    if (TARGET > URLnorm)
    TARGET = URLnorm;
    end
    if (TARGET < LRLnorm)
    TARGET = LRLnorm;
    end
  (default) -> START
  START -> SLOPE_CALCULATION
  RATE_CALCULATION -> SLOPE_CALCULATION : after(100, msec)
  SLOPE_CALCULATION -> RATE_CALCULATION : after(1, msec)
  data: LRL input uint16; URL input uint16; THRESH input uint16; RF input uint16; REACTION_TIME input uint16; RECOVERY_TIME input uint16; step_recovery local uint16; step_reaction local uint16; RATE local uint16; OUTPUT_RATE output uint16; TARGET local uint16; LRLnorm local uint16; URLnorm local uint16; slope local uint16; MSR input uint16; ACTIVITY local uint16; ACTIVITYIN input
